simulink subsystem "T0_from_date"  (R2022a)
settings: Solver=VariableStepAuto  StartTime=0.0  StopTime=10.0  RelTol=1e-3
settings Model: Creator=samuel  LastModifiedBy=samuel

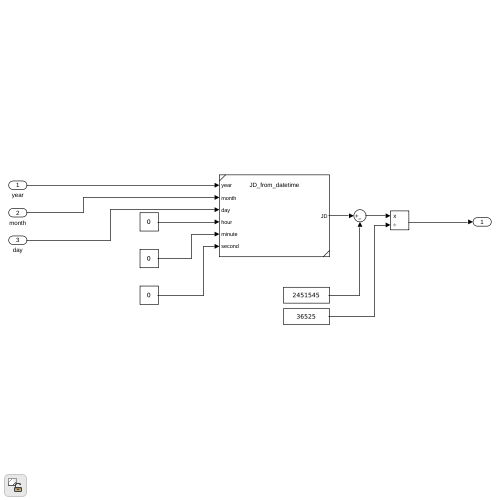
[thumbnail: Simulink's stored preview of the top-level diagram]
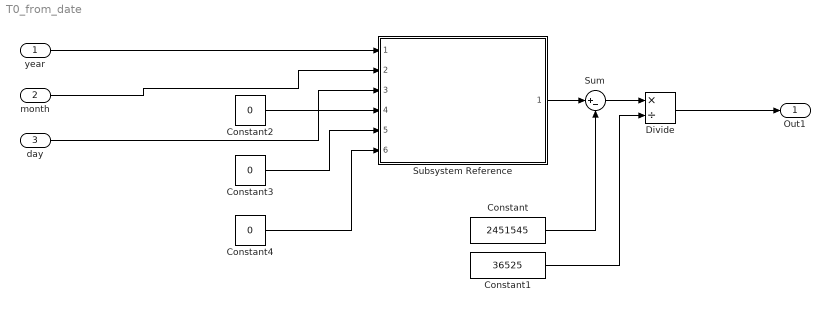
== system T0_from_date ==
  year : Inport
  month : Inport  Port=2
  day : Inport  Port=3
  Constant : Constant  Value=2451545
  Constant1 : Constant  Value=36525
  Constant2 : Constant  Value=0
  Constant3 : Constant  Value=0
  Constant4 : Constant  Value=0
  Divide : Product  Inputs=*/
  Subsystem Reference : Subsystem  ReferencedSubsystem=JD_from_datetime
  Sum : Sum  Inputs=|+-
  Out1 : Outport
  wires:
  Constant3/1 -> Subsystem Reference/5
  Subsystem Reference/1 -> Sum/1
  Constant/1 -> Sum/2
  Constant1/1 -> Divide/2
  Constant2/1 -> Subsystem Reference/4
  Constant4/1 -> Subsystem Reference/6
  Divide/1 -> Out1/1
  year/1 -> Subsystem Reference/1
  day/1 -> Subsystem Reference/3
  Sum/1 -> Divide/1
  month/1 -> Subsystem Reference/2
